simulink model "Sim_Model_2ndODE_ex2"  (Simulink 8.0)
settings: Solver=ode45  StartTime=0.0  StopTime=10.0  RelTol=1e-3
undefined symbols (not defined in the file or in its folder): K1, K2
settings Model: Creator=David  LastModifiedBy=David
settings DataIOCC: SignalLoggingSaveFormat=ModelDataLogs
settings DebuggingCC: FcnCallInpInsideContextMsg=UseLocalSettings
settings GRTTargetCC: CombineOutputUpdateFcns=off  GRTInterface=on

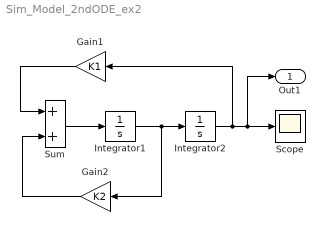
== system Sim_Model_2ndODE_ex2 ==
  Gain1 : Gain  Gain=K1
  Gain2 : Gain  Gain=K2
  Integrator1 : Integrator
  Integrator2 : Integrator  InitialCondition=2
  Scope : Scope
  Sum : Sum
  Out1 : Outport
  wires:
  Sum/1 -> Integrator1/1
  Gain1/1 -> Sum/1
  Integrator1/1 -> Gain2/1, Integrator2/1
  Integrator2/1 -> Gain1/1, Out1/1, Scope/1
  Gain2/1 -> Sum/2
